simulink model "Lab9_zadanie1"  (R2017a)
settings: Solver=FixedStepAuto  StartTime=0.0  StopTime=20  FixedStep=0.01  RelTol=1e-3
values from neighbouring files (symbols this model uses):
  a = (P1y - P2y) / (P1x - P2x)    (= 0.457251908397)    [Lab4.m]    (also in Lab8.m = 10; Lab9.m = 0.01)
  B = (pi*R2*R2)/(3*H2*H2)    (= 0.00337009933323)    [Lab2.m]    (also in Lab8.m = deltah20max / k; Lab9.m = 0.4; ModelDataNonlinear.m)
  delta = 0.005    [Lab9.m]
  ks = 10    [Lab9.m]
  Tm = Ts/(kr*ks)    (= 26.2488954345)    [Lab9.m]
  Ts = Ti    (= 17.823)    [Lab9.m]
settings Model: Creator=ishiguro  LastModifiedBy=ishiguro

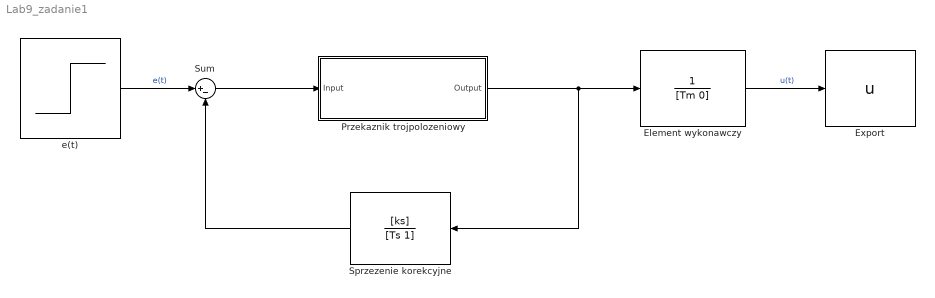
== system Lab9_zadanie1 ==
  Element wykonawczy : TransferFcn  Denominator=[Tm 0]
  Export : ToWorkspace  VariableName=u  SaveFormat=Timeseries  SampleTime=-1
  "Przekaznik trojpolozeniowy " : Subsystem
  Sprzezenie korekcyjne : TransferFcn  Numerator=[ks]  Denominator=[Ts 1]
  Sum : Sum  Inputs=|+-
  e(t) : Step  Time=0  SampleTime=0
  wires:
  e(t)/1 -> Sum/1  "e(t)"
  Sprzezenie korekcyjne/1 -> Sum/2
  Element wykonawczy/1 -> Export/1  "u(t)"
  "Przekaznik trojpolozeniowy "/1(Output) -> Element wykonawczy/1, Sprzezenie korekcyjne/1
  Sum/1 -> "Przekaznik trojpolozeniowy "/1("Input ")

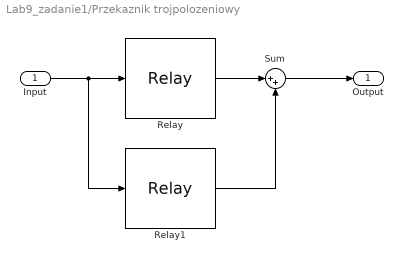
== system Lab9_zadanie1/Przekaznik trojpolozeniowy  ==
  "Input " : Inport
  Relay : Relay  OnSwitchValue=-a  OffSwitchValue=-a-delta  OnOutputValue=0  OffOutputValue=-B
  Relay1 : Relay  OnSwitchValue=a+delta  OffSwitchValue=a  OnOutputValue=B
  Sum : Sum  Inputs=|++
  Output : Outport
  wires:
  "Input "/1 -> Relay1/1, Relay/1
  Relay1/1 -> Sum/2
  Relay/1 -> Sum/1
  Sum/1 -> Output/1
